simulink model "mass_spring_damper_model"  (R2025a)
settings: Solver=FixedStepAuto  StartTime=0.0  StopTime=inf  FixedStep=0.001  RelTol=1e-3
values from neighbouring files (symbols this model uses):
  c = 0.008    [data_clean.m]
  ext_force = F_gravity    (= 3177.3546)    [data_clean.m]
  init = 30    [data_clean.m]
  k = 29.32750224    [data_clean.m]
  m = m_plate + (5 * m_nut)    (= 0.324)    [data_clean.m]
libraries: instrumentseriallib x2, stmutilitieslib x1
settings Model: Creator=User  LastModifiedBy=User

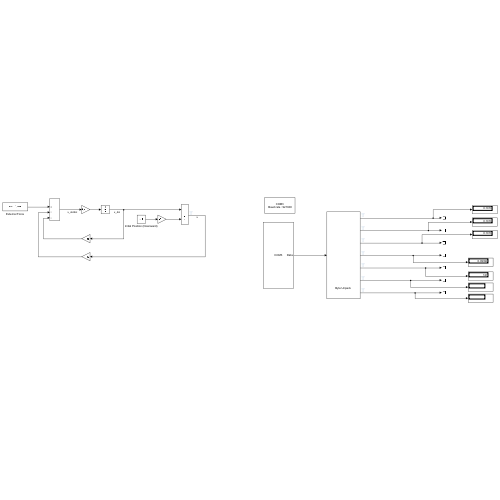
[thumbnail: Simulink's stored preview of the top-level diagram]
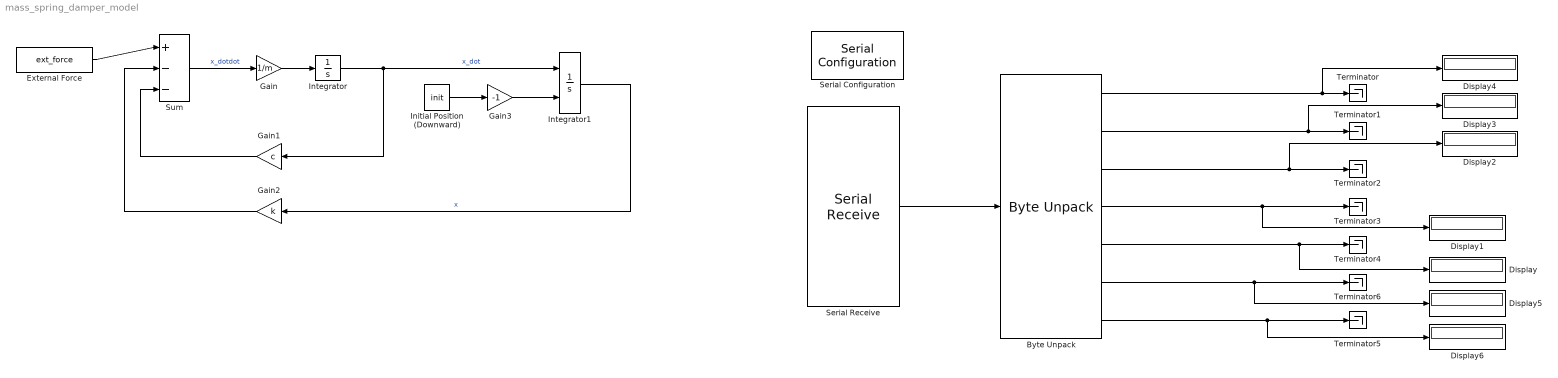
== system mass_spring_damper_model ==
  Byte Unpack : stmutilitieslib/Byte Unpack  dimensions={1, 1, 1, 1, 1, 1, 1}  datatypes={'single', 'single', 'single', 'single', 'single', 'single', 'uint8'}  byteAlign=1  blockPlatform=stm32f4discovery
  Display{,1..6} (7 alike) : Display
  External Force : Constant  Value=ext_force
  Gain : Gain  Gain=1/m
  Gain1 : Gain  Gain=c
  Gain2 : Gain  Gain=k
  Gain3 : Gain  Gain=-1
  Initial Position (Downward) : Constant  Value=init
  Integrator : Integrator
  Integrator1 : Integrator  InitialConditionSource=external
  Serial Configuration : instrumentseriallib/Serial Configuration  Priority=-200000  PortSel=COM3  Port=COM3  ComPort=COM3  BaudRate=921600  DataBits=8  Parity=none  StopBits=1  ByteOrder=little-endian  FlowControl=none  Timeout=10  SimulateUsing=Interpreted execution  BlockInModel=on  aMode=1
      settings: LibrarySourceBlock=embeddedtargetslib/Host Communication/Serial Configuration
  Serial Receive : instrumentseriallib/Serial Receive  Priority=1  PortSel=COM3  Port=COM3  ComPort=COM3  DataType=uint8  SaveDataType=uint8  ToggleHeader=on  Header=[205 171]  ToggleDataSize=on  DataSize=[25 1]  ToggleTerminator=off  Terminator=<none>  CustomTerminator=[]  InputFormat=Column major  EnableBlockingMode=on  ActionDataUnavailable=Output last received value  ActionWhenDataUnavailable=Output last received value  CustomValue=0  SampleTime=0.001  SimulateUsing=Interpreted execution  BlockInModel=on  aMode=1  LibraryInUse=instrumentlib
      settings: LibrarySourceBlock=embeddedtargetslib/Host Communication/Serial Receive
  Sum : Sum  Inputs=|+--
  Terminator{,1..6} (7 alike) : Terminator
  wires:
  Serial Receive/1 -> Byte Unpack/1
  Byte Unpack/1 -> Display4/1, Terminator/1
  Sum/1 -> Gain/1  "x_dotdot"
  Gain/1 -> Integrator/1
  Integrator/1 -> Gain1/1, Integrator1/1  "x_dot"
  Gain1/1 -> Sum/3
  Integrator1/1 -> Gain2/1  "x"
  Gain2/1 -> Sum/2
  External Force/1 -> Sum/1
  Initial Position (Downward)/1 -> Gain3/1
  Gain3/1 -> Integrator1/2
  Byte Unpack/2 -> Display3/1, Terminator1/1
  Byte Unpack/3 -> Display2/1, Terminator2/1
  Byte Unpack/4 -> Display1/1, Terminator3/1
  Byte Unpack/5 -> Terminator4/1, Display/1
  Byte Unpack/6 -> Display5/1, Terminator6/1
  Byte Unpack/7 -> Display6/1, Terminator5/1
